simulink model "testing"  (R2020a)
settings: Solver=VariableStepAuto  StartTime=0.0  StopTime=10.0  RelTol=1e-3
settings Model: Creator=Makar  LastModifiedBy=Makar

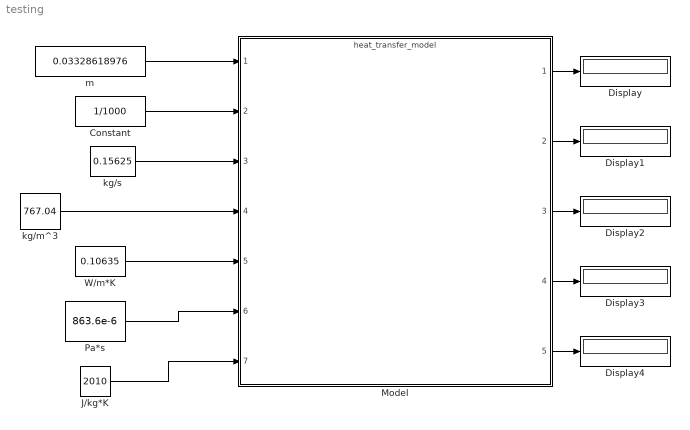
== system testing ==
  Constant : Constant  Value=1/1000
  Display{,1..4} (5 alike) : Display
  J/kg*K : Constant  Value=2010
  Model : ModelReference  ModelNameDialog=heat_transfer_model.slx  SimulationMode=Normal  ModelReferenceVersion=1.9
  Pa*s : Constant  Value=863.6e-6
  W/m*K : Constant  Value=0.10635
  kg/m^3 : Constant  Value=767.04
  kg/s : Constant  Value=0.15625
  m : Constant  Value=0.03328618976
  wires:
  m/1 -> Model/1
  Constant/1 -> Model/2
  kg/s/1 -> Model/3
  kg/m^3/1 -> Model/4
  W/m*K/1 -> Model/5
  Pa*s/1 -> Model/6
  J/kg*K/1 -> Model/7
  Model/1 -> Display/1
  Model/2 -> Display1/1
  Model/3 -> Display2/1
  Model/4 -> Display3/1
  Model/5 -> Display4/1
